simulink model "prob2"  (R2020b)
settings: Solver=VariableStepAuto  StartTime=0.0  StopTime=10.0  RelTol=1e-3
undefined symbols (not defined in the file): b, k1, k2, M1, M2
settings Model: Creator=nadee  LastModifiedBy=nadee

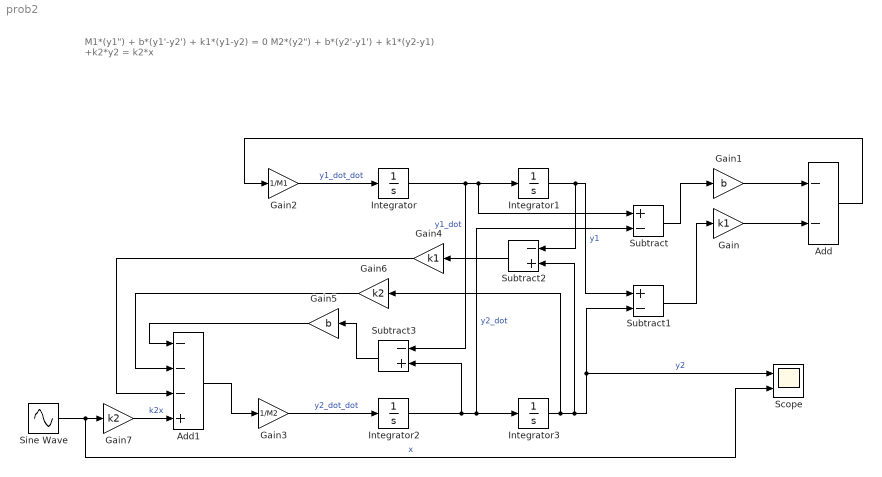
== system prob2 ==
  note: M1*(y1") + b*(y1'-y2') + k1*(y1-y2) = 0
      | M2*(y2") + b*(y2'-y1') + k1*(y2-y1) +k2*y2 = k2*x
  Add : Sum  Inputs=--
  Add1 : Sum  Inputs=---+
  Gain : Gain  Gain=k1
  Gain1 : Gain  Gain=b
  Gain2 : Gain  Gain=1/M1
  Gain3 : Gain  Gain=1/M2
  Gain4 : Gain  Gain=k1
  Gain5 : Gain  Gain=b
  Gain6 : Gain  Gain=k2
  Gain7 : Gain  Gain=k2
  Integrator{,1..3} (4 alike) : Integrator
  Scope : Scope  NumInputPorts=2
  Sine Wave : Sin  SampleTime=0
  Subtract : Sum  Inputs=+-
  Subtract1 : Sum  Inputs=+-
  Subtract2 : Sum  Inputs=-+
  Subtract3 : Sum  Inputs=-+
  wires:
  Integrator1/1 -> Subtract2/1, Subtract1/1  "y1"
  Integrator/1 -> Subtract3/1, Subtract/1, Integrator1/1  "y1_dot"
  Gain2/1 -> Integrator/1  "y1_dot_dot"
  Gain3/1 -> Integrator2/1  "y2_dot_dot"
  Integrator2/1 -> Subtract3/2, Integrator3/1, Subtract/2  "y2_dot"
  Integrator3/1 -> Gain6/1, Subtract2/2, Scope/1, Subtract1/2  "y2"
  Add/1 -> Gain2/1
  Subtract/1 -> Gain1/1
  Subtract1/1 -> Gain/1
  Gain/1 -> Add/2
  Gain1/1 -> Add/1
  Add1/1 -> Gain3/1
  Subtract2/1 -> Gain4/1
  Subtract3/1 -> Gain5/1
  Gain4/1 -> Add1/3
  Gain6/1 -> Add1/2
  Gain5/1 -> Add1/1
  Gain7/1 -> Add1/4  "k2x"
  Sine Wave/1 -> Scope/2, Gain7/1  "x"
